simulink model "Assignment_TestGen11"  (R2017b)
settings: Solver=FixedStepDiscrete  StartTime=0.0  StopTime=10.0  RelTol=1e-3
settings Model: Creator=hbourbou  LastModifiedBy=hbourbou
settings DebuggingCC: ParameterOverflowMsg=none

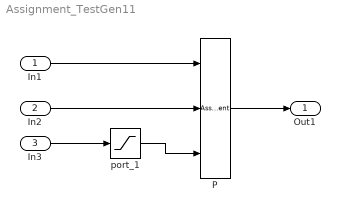
== system Assignment_TestGen11 ==
  In1 : Inport  OutDataTypeStr=uint16  PortDimensions=[3 3 3]
  In2 : Inport  Port=2  OutDataTypeStr=uint16  PortDimensions=[3 2 2]
  In3 : Inport  Port=3  OutMin=1  OutMax=2
  P : Assignment  NumberOfDimensions=3  DiagnosticForDimensions=Warning  IndexOptions=Assign all,Index vector (dialog),Index vector (port)  Indices=[],[1,2],[]  OutputSizes=,,
  port_1 : Saturate  UpperLimit=2  LowerLimit=1
  Out1 : Outport
  wires:
  In1/1 -> P/1
  In2/1 -> P/2
  port_1/1 -> P/3
  In3/1 -> port_1/1
  P/1 -> Out1/1
